simulink model "state_trans"  (R2023b)
settings: Solver=VariableStepAuto  StartTime=0.0  StopTime=10  RelTol=1e-3
values from neighbouring files (symbols this model uses):
  A1 = double(trans_A)    [test.m]
  A2 = double(trans_A)    [test.m]
  A3 = double(trans_A)    [test.m]
  A4 = double(trans_A)    [test.m]
  A5 = double(trans_A)    [test.m]
  B1 = double(trans_B)    [test.m]
  B2 = double(trans_B)    [test.m]
  B3 = double(trans_B)    [test.m]
  B4 = double(trans_B)    [test.m]
  B5 = double(trans_B)    [test.m]
  K1 = KK    [test.m]
  K2 = KK    [test.m]
  K3 = KK    [test.m]
  K4 = KK    [test.m]
  K5 = KK    [test.m]
  trans_C = eye(10)    [test.m]
  trans_D = zeros(10,4)    [test.m]
libraries: simulink x1
settings Model: Creator=84103  LastModifiedBy=84103

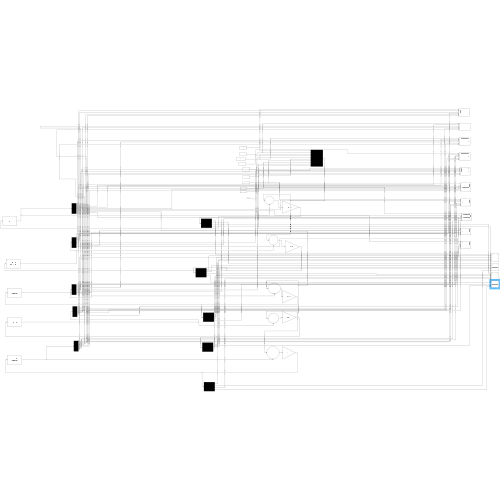
[thumbnail: Simulink's stored preview of the top-level diagram]
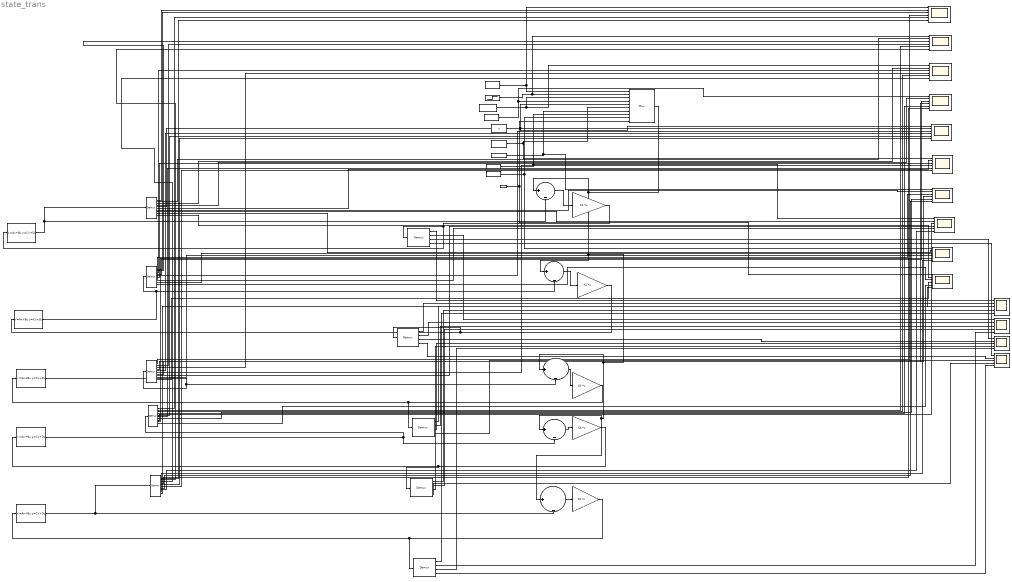
== system state_trans ==
  Constant{1..8} (8 alike) : Constant  Value=0
  Demux{,3,5,7,9} (5 alike) : Demux  Outputs=10
  Demux{1..2,4,6,8} (5 alike) : Demux
  Gain : Gain  Gain=K1  Multiplication=Matrix(K*u) (u vector)
  Gain1 : Gain  Gain=K2  Multiplication=Matrix(K*u) (u vector)
  Gain2 : Gain  Gain=K3  Multiplication=Matrix(K*u) (u vector)
  Gain3 : Gain  Gain=K4  Multiplication=Matrix(K*u) (u vector)
  Gain4 : Gain  Gain=K5  Multiplication=Matrix(K*u) (u vector)
  Mux : Mux  Inputs=10
  Ramp : simulink/Sources/Ramp  slope=2  start=0.1  InitialOutput=0
  Scope{,1..9} (10 alike) : Scope  NumInputPorts=6
  Scope{10..13} (4 alike) : Scope  NumInputPorts=5
  State-Space : StateSpace  A=A1  B=B1  C=trans_C  D=trans_D  InitialCondition=[0;0;0;0;0;0;0;0;0;0]
  State-Space1 : StateSpace  A=A2  B=B2  C=trans_C  D=trans_D  InitialCondition=[0;0;0;0;0;0;0;0;0;0]
  State-Space2 : StateSpace  A=A3  B=B3  C=trans_C  D=trans_D  InitialCondition=[0;0;0;0;0;0;0;0;0;0]
  State-Space3 : StateSpace  A=A4  B=B4  C=trans_C  D=trans_D  InitialCondition=[0;0;0;0;0;0;0;0;0;0]
  State-Space4 : StateSpace  A=A5  B=B5  C=trans_C  D=trans_D  InitialCondition=[0;0;0;0;0;0;0;0;0;0]
  Step : Step  Time=0.1  After=2  SampleTime=0
  Sum{,1..4} (5 alike) : Sum  Inputs=|+-
  wires:
  State-Space/1 -> Demux/1, Sum/2
  Gain/1 -> State-Space/1, Demux1/1
  Mux/1 -> Sum1/1, Sum4/1, Sum3/1, Sum2/1, Sum/1
  Sum/1 -> Gain/1
  Demux1/1 -> Scope10/1
  Demux1/2 -> Scope11/1
  Demux1/3 -> Scope12/1
  Demux1/4 -> Scope13/1
  State-Space1/1 -> Sum1/2, Demux3/1
  Sum1/1 -> Gain1/1
  Gain1/1 -> State-Space1/1, Demux2/1
  State-Space2/1 -> Sum2/2, Demux5/1
  Sum2/1 -> Gain2/1
  Gain2/1 -> Demux4/1, State-Space2/1
  Ramp/1 -> Mux/1, Scope/1
  Step/1 -> Mux/2, Scope1/1
  Constant8/1 -> Mux/3, Scope2/1
  Constant1/1 -> Scope3/1, Mux/4
  Constant2/1 -> Scope4/1, Mux/5
  Constant3/1 -> Mux/6, Scope5/1
  Constant5/1 -> Scope7/1, Mux/8
  Constant6/1 -> Scope8/1, Mux/9
  Constant7/1 -> Scope9/1, Mux/10
  Constant4/1 -> Mux/7, Scope6/1
  Demux/1 -> Scope/2
  Demux/2 -> Scope1/2
  Demux/3 -> Scope2/2
  Demux/4 -> Scope3/2
  Demux/5 -> Scope4/2
  Demux/6 -> Scope5/2
  Demux/7 -> Scope6/2
  Demux/8 -> Scope7/2
  Demux/9 -> Scope8/2
  Demux/10 -> Scope9/2
  Demux3/1 -> Scope/3
  Demux3/2 -> Scope1/3
  Demux3/3 -> Scope2/3
  Demux3/4 -> Scope3/3
  Demux3/5 -> Scope4/3
  Demux3/6 -> Scope5/3
  Demux3/7 -> Scope6/3
  Demux3/8 -> Scope7/3
  Demux3/9 -> Scope8/3
  Demux3/10 -> Scope9/3
  Demux5/1 -> Scope/4
  Demux5/2 -> Scope1/4
  Demux5/3 -> Scope2/4
  Demux5/4 -> Scope3/4
  Demux5/5 -> Scope4/4
  Demux5/6 -> Scope5/4
  Demux5/7 -> Scope6/4
  Demux5/8 -> Scope7/4
  Demux5/9 -> Scope8/4
  Demux5/10 -> Scope9/4
  Demux2/1 -> Scope10/2
  Demux4/1 -> Scope10/3
  Demux2/2 -> Scope11/2
  Demux4/2 -> Scope11/3
  Demux2/3 -> Scope12/2
  Demux4/3 -> Scope12/3
  Demux2/4 -> Scope13/2
  Demux4/4 -> Scope13/3
  State-Space3/1 -> Demux7/1, Sum3/2
  Sum3/1 -> Gain3/1
  Gain3/1 -> Demux6/1, State-Space3/1
  Demux6/1 -> Scope10/4
  Demux6/2 -> Scope11/4
  Demux6/3 -> Scope12/4
  Demux6/4 -> Scope13/4
  Demux7/1 -> Scope/5
  Demux7/2 -> Scope1/5
  Demux7/3 -> Scope2/5
  Demux7/4 -> Scope3/5
  Demux7/5 -> Scope4/5
  Demux7/6 -> Scope5/5
  Demux7/7 -> Scope6/5
  Demux7/8 -> Scope7/5
  Demux7/9 -> Scope8/5
  Demux7/10 -> Scope9/5
  State-Space4/1 -> Sum4/2, Demux9/1
  Sum4/1 -> Gain4/1
  Gain4/1 -> Demux8/1, State-Space4/1
  Demux8/1 -> Scope10/5
  Demux8/2 -> Scope11/5
  Demux8/3 -> Scope12/5
  Demux8/4 -> Scope13/5
  Demux9/1 -> Scope/6
  Demux9/2 -> Scope1/6
  Demux9/3 -> Scope2/6
  Demux9/4 -> Scope3/6
  Demux9/5 -> Scope4/6
  Demux9/6 -> Scope5/6
  Demux9/7 -> Scope6/6
  Demux9/8 -> Scope7/6
  Demux9/9 -> Scope8/6
  Demux9/10 -> Scope9/6
